simulink library "svm_lib"  (Simulink 8.6)
settings: Solver=VariableStepAuto  StartTime=0.0  StopTime=10.0  RelTol=1e-3
values from neighbouring files (symbols this model uses):
  My_3D = ([eye(6) -eye(6)])    [svm_buildLinearControllers.m]    (also in svm_setup.m = [-eye(6) eye(6)])
  turbulence2loadfactors = blkdiag(T_w2nx, T_w2nz)    [svm_buildLinearControllers.m]
  uavsim = loaded.uavsim    [svm_sandbox.m]
undefined symbols (not defined in the file or in its folder): dt, F, fflib_delay_c2d, Light, mask_p0_NED, mask_v0_NED, MIL, postracking, svm, uavsimblockset_cartesianToAngle
libraries: svm_lib x9, simulink_extras x8, aerolibtransform2 x3, formationFlyingBlockset x2, uavsimBlockset_Cularis_Aerandpropulsion x1, uavsimBlockset_ElectricPropulsion x1, aerolibwind2 x1, aerolibgravity2 x1, uavsimBlockset_VectorNorm x1, uavsimBlockset_UAV3DInterface x1
(part 2 of 3)

== system svm_lib/vector2bus u ==
  u_bus : Inport  PortDimensions=3
  Bus Object Bus Creator : BusCreator  Inputs=1  OutDataTypeStr=Bus: svm_bus_u  mask(BUS OBJECT Bus Creator){busType=Bus: svm_bus_u}
      mask prompts: busType "Bus Type"
      mask help:
      | Provides users the cabability to painlessly, instantly customize bus creators of output data type 'Bus:' by selecting the bus object type from a drop down menu dynamically populated by bus objects in the workspace.
      |
      | After pressing the "Apply Selection" button signal lines into the creator are populated and named with the elements in the chosen bus saving the user from having to recall and fill out signal line names.
      |
      | NOTE that when copying a Bus Object Bus Creator from your locked Library the link to the Library is automatically broken. This saves the user from having to Unlock Links To Library (From the Library menu.), Disable Link and finally Break Link (Both from the Model menu.) for every placed instance of the block.
      settings: AttributesFormatString=%<OutDataTypeStr>  CopyFcn=set_param(gcb, 'LinkStatus', 'none')
      mask TypeOptions busType: Bus: Acceleration | Bus: Aero | Bus: Airframe | Bus: Attitude | Bus: CMD | Bus: Environment | Bus: FlightGearData | Bus: Kinematics | Bus: Position | Bus: RotationalAcceleration | Bus: RotationalVelocity | Bus: Velocity | Bus: svm_bus_d_exo | Bus: svm_bus_u | Bus: svm_bus_x | Bus: svm_bus_xi
      mask Callback busType:
      | % Using variable names terminated with "_BOBC" to lessen the chances of
      | % collisions with existing workspace variables.
      | 
      | % Get the current block handle and mask handle.
      | handleCreator_BOBC = gcbh;
      | maskObj_BOBC       = Simulink.Mask.get(gcb);
      | 
      | % Get a list of variables in the workspace in order to search for the '1x1
      | % Bus' types.
      | wsVars_BOBC = whos;
      | 
      | % Reset the 'TypeOptions' bus list in case some '1x1 Bus' types have been
      | % deleted from or added to the workspace.
      | maskObj_BOBC.Parameters.TypeOptions = {'<empty>'};
      | 
      | % Reset the bus count.
      | busCount_BOBC = 0;
      | 
      | for index_BOBC = 1:length(wsVars_BOBC)
      | 
      |    % If the variable is a bus object...
      |    if strcmp(wsVars_BOBC(index_BOBC).class, 'Simulink.Bus')
      | 
      |       busCount_BOBC = busCount_BOBC + 1;
      | 
      |       % ... add it to the TypeOptions of the mask.
      |       maskObj_BOBC.Parameters.TypeOptions(busCount_BOBC) = ...
      |                                                            ...
      |                                  {['Bus: ', wsVars_BOBC(index_BOBC).name]};
      |    end
      | end
      | 
      | if busCount_BOBC == 0
      | 
      |    % If there are NO bus objects in the workspace then provide a warning
      |    % popup...
      |    warndlg('There are currently no bus objects in the workspace - you have no use for this block. Use a normal Bus Creator instead.')
      | 
      |    % ... and do nothing.
      | elseif ~strcmp(get_param(handleCreator_BOBC, 'OutDataTypeStr'), 'Inherit: auto')
      | 
      |    % If the currently selected bus data type ('OutDataTypeStr') is not
      |    % 'Inherit: auto' (i.e., if we are reopening the mask.) then get the
      |    % current 'OutDataTypeStr' and 'maskVal.' ('maskVal' is the selected
      |    % 'TypeOptions' list member.)
      |    outDatStr_BOBC = get_param(handleCreator_BOBC, 'OutDataTypeStr');
      |    maskVal_BOBC   = get_param(handleCreator_BOBC, 'MaskValues');
      | 
      |    if ~strcmp(outDatStr_BOBC, maskVal_BOBC{1})
      | 
      |       % Upon re-opening the mask if the default 'TypeOptions' list member
      |       % (The first one.) contained in 'maskVal' does not match the
      |       % currently selected bus data type ('OutDataTypeStr') then set the
      |       % 'TypeOptions' list member to the selected bus data type. (Cuts down
      |       % on confusion to have the displayed list member match the selected
      |       % bus data type rather than the first entry.)
      |       set_param(handleCreator_BOBC, 'MaskValues', {outDatStr_BOBC});
      |    end
      | end
      | 
      | % Clean up the workspace.
      | clear  handleCreator_BOBC  maskObj_BOBC     wsVars_BOBC ...
      |             busCount_BOBC    index_BOBC  outDatStr_BOBC ...
      |              maskVal_BOBC
      mask DialogControl applyMOCBSelection Prompt: Apply Selection
      mask DialogControl applyMOCBSelection Callback:
      | % Using variable names terminated with "_BOBC" to lessen the chances of
      | % collisions with existing workspace variables.
      | 
      | % Get the current block, current block handle and mask handle.
      | currentBlock_BOBC  = gcb;
      | handleCreator_BOBC = gcbh;
      | 
      | % Get the desired bus type...
      | desiredBusType_BOBC = get_param(handleCreator_BOBC, 'busType');
      | 
      | % ... and set the 'OutDataTypeStr' to it.
      | set_param(handleCreator_BOBC, 'OutDataTypeStr', desiredBusType_BOBC);
      | 
      | %% First delete any existing lines on the port.
      | % Get the line handles.
      | lh_BOBC = get_param(handleCreator_BOBC, 'LineHandles');
      | 
      | % If any lines exist (Non- -1 line handles.), delete them and start over.
      | if max(lh_BOBC.Inport > 0)
      | 
      |    for index_BOBC = 1:length(lh_BOBC.Inport)
      | 
      |       if lh_BOBC.Inport(index_BOBC) > 0
      | 
      |          delete_line(lh_BOBC.Inport(index_BOBC))
      |       end
      |    end
      | end
      | 
      | %% Then work on adding new lines.
      | 
      | % Get the block path for 'add_line' function.
      | blockPath_BOBC = get_param(handleCreator_BOBC, 'Parent');
      | 
      | % Get the newly selected bus type ('OutDataTypeStr')...
      | mocbBusType_BOBC = get_param(currentBlock_BOBC, 'OutDataTypeStr');
      | 
      | % ... and parse off "Bus: " so the string of the desired bus contained in
      | % 'OutDataTypeStr' matches the raw workspace bus names.
      | mocbBusType_BOBC = mocbBusType_BOBC(6:end);
      | 
      | % Then evaluate the string containing the workspace bus name which will
      | % load the desired bus parameters.
      | busParams_BOBC = eval(mocbBusType_BOBC);
      | 
      | % From the parameters grab the number of lines to add.
      | numLines_BOBC = length(busParams_BOBC.Elements);
      | 
      | % Set the number of inputs of the masked bus creator to the number of lines
      | % to add.
      | set_param(handleCreator_BOBC, 'Inputs', num2str(numLines_BOBC));
      | 
      | % Get (Inputs.) port handles so we can grab the positions of them.
      | ph_BOBC = get_param(handleCreator_BOBC, 'PortHandles');
      | 
      | for index_BOBC = 1:numLines_BOBC
      | 
      |    % Get the position of input port number 'index_BOBC'.
      |    portPos_BOBC = get_param(ph_BOBC.Inport(index_BOBC), 'Position');
      | 
      |    % Add a line from 50 pixels left of the port position to the port
      |    % position. (This must be done because it's the lines that get named,
      |    % not the port positions.)
      |    portLine_BOBC = add_line(blockPath_BOBC, [portPos_BOBC - [50 0]; portPos_BOBC]);
      | 
      |    % Rename the new line to the bus 'index_BOBC-st/nd/rd/th' element name.
      |    set_param(portLine_BOBC, 'Name', busParams_BOBC.Elements(index_BOBC).Name)
      | end
      | 
      | %% Cleanup the workspace.
      | clear    currentBlock_BOBC  handleCreator_BOBC      index_BOBC ...
      |        desiredBusType_BOBC             lh_BOBC  blockPath_BOBC ...
      |           mocbBusType_BOBC      busParams_BOBC   numLines_BOBC ...
      |                    ph_BOBC        portPos_BOBC   portLine_BOBC
  u_vector : Outport
  wires:
  u_bus/1 -> Bus Object Bus Creator/1  "n"
  Bus Object Bus Creator/1 -> u_vector/1

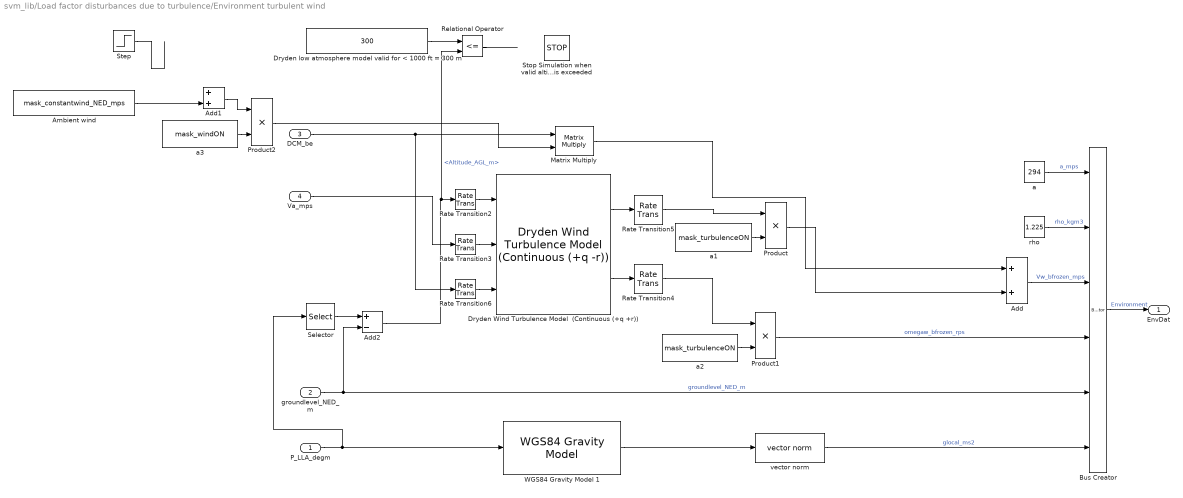
== system svm_lib/Load factor disturbances due to turbulence/Environment turbulent wind ==
  P_LLA_degm : Inport
  groundlevel_NED_m : Inport  Port=2
  DCM_be : Inport  Port=3
  Va_mps : Inport  Port=4
  Add : Sum
  Add1 : Sum
  Add2 : Sum  Inputs=+-
  Ambient wind : Constant  Value=mask_constantwind_NED_mps
  Bus Creator : BusCreator  Inputs=6  OutDataTypeStr=Bus: Environment  NonVirtualBus=on
  Dryden Wind Turbulence Model  (Continuous (+q +r)) : aerolibwind2/Dryden Wind Turbulence Model  (Continuous (+q -r))  units=Metric (MKS)  spec=MIL-F-8785C  model=Discrete Dryden (+q -r)  W20=norm(mask_constantwind_NED_mps)  Wdeg=rad2deg(uavsimblockset_cartesianToAngle(mask_constantwind_NED_mps(1), mask_constantwind_NED_mps(2)))  TurbProb=10^-2 - Light  L_high=533.4  Wingspan=mask_wingspan  ts=0.1  Seed=eval(svm.turbulenceseed)  T_on=on
  Dryden low atmosphere model valid for < 1000 ft = 300 m : Constant  Value=300
  Matrix Multiply : Product  Multiplication=Matrix(*)
  Product : Product  RndMeth=Zero
  Product1 : Product  RndMeth=Zero
  Product2 : Product  RndMeth=Zero
  Rate Transition2 : RateTransition  OutPortSampleTime=0.1
  Rate Transition3 : RateTransition  OutPortSampleTime=0.1
  Rate Transition4 : RateTransition  OutPortSampleTime=0
  Rate Transition5 : RateTransition  OutPortSampleTime=0
  Rate Transition6 : RateTransition  OutPortSampleTime=0.1
  Relational Operator : RelationalOperator  Operator=<=  OutDataTypeStr=boolean
  Selector : Selector  InputPortWidth=3  IndexOptions=Index vector (dialog)  Indices=3  OutputSizes=1
  Step : Step  Time=10  After=[0 0 1]  SampleTime=0
  Stop Simulation when valid altitude is exceeded : Stop
  WGS84 Gravity Model 1 : aerolibgravity2/WGS84 Gravity Model   model=WGS84 Taylor Series  units=Metric (MKS)  no_atmos=on  precessing=on  jd_loc=off  month=October  day=10  year=2004  no_centrifugal=on  action=Warning
  a : Constant  Value=294
  a1 : Constant  Value=mask_turbulenceON
  a2 : Constant  Value=mask_turbulenceON
  a3 : Constant  Value=mask_windON
  "rho " : Constant  Value=1.225
  vector norm : uavsimBlockset_VectorNorm/vector norm
  EnvDat : Outport  OutDataTypeStr=Bus: Environment
  wires:
  Step/1 -> ?
  Add1/1 -> Product2/1
  Product2/1 -> Matrix Multiply/2
  a3/1 -> Product2/2
  Relational Operator/1 -> ?
  Dryden low atmosphere model valid for < 1000 ft = 300 m/1 -> Relational Operator/1
  Product1/1 -> Bus Creator/4  "omegaw_bfrozen_rps"
  a2/1 -> Product1/2
  a1/1 -> Product/2
  Product/1 -> Add/2
  Dryden Wind Turbulence Model  (Continuous (+q +r))/2 -> Rate Transition4/1
  P_LLA_degm/1 -> WGS84 Gravity Model 1/1, Selector/1
  groundlevel_NED_m/1 -> Add2/2, Bus Creator/5  "groundlevel_NED_m"
  WGS84 Gravity Model 1/1 -> vector norm/1
  Bus Creator/1 -> EnvDat/1  "Environment"
  "rho "/1 -> Bus Creator/2  "rho_kgm3"
  a/1 -> Bus Creator/1  "a_mps"
  Add/1 -> Bus Creator/3  "Vw_bfrozen_mps"
  vector norm/1 -> Bus Creator/6  "glocal_ms2"
  Add2/1 -> Rate Transition2/1, Relational Operator/2  "<Altitude_AGL_m>"
  Va_mps/1 -> Rate Transition3/1
  DCM_be/1 -> Matrix Multiply/1, Rate Transition6/1
  Ambient wind/1 -> Add1/2
  Dryden Wind Turbulence Model  (Continuous (+q +r))/1 -> Rate Transition5/1
  Matrix Multiply/1 -> Add/1
  Rate Transition4/1 -> Product1/1
  Rate Transition5/1 -> Product/1
  Selector/1 -> Add2/1
  Rate Transition2/1 -> Dryden Wind Turbulence Model  (Continuous (+q +r))/1
  Rate Transition3/1 -> Dryden Wind Turbulence Model  (Continuous (+q +r))/2
  Rate Transition6/1 -> Dryden Wind Turbulence Model  (Continuous (+q +r))/3

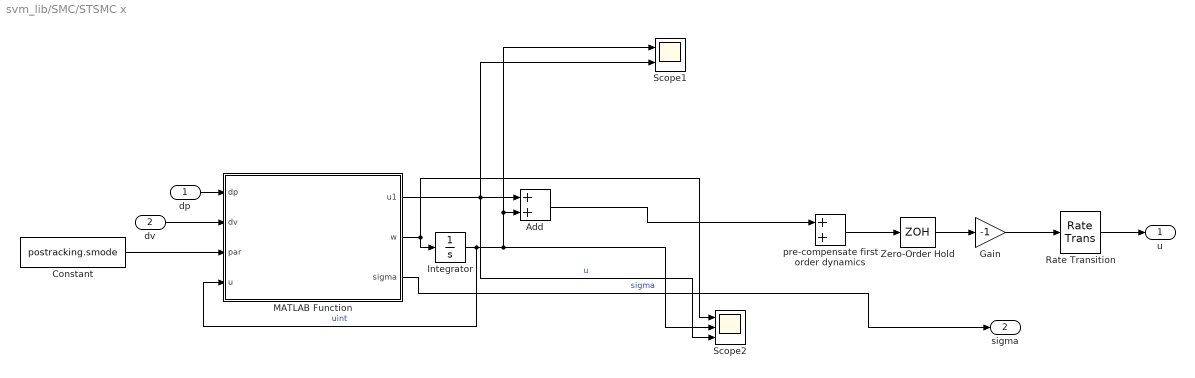
== system svm_lib/SMC/STSMC x ==
  dp : Inport
  dv : Inport  Port=2
  Add : Sum
  Constant : Constant  Value=postracking.smode  OutDataTypeStr=Bus: slBus1
  Gain : Gain  Gain=-1
  Integrator : Integrator
  MATLAB Function : MATLAB Function  TreatAsAtomicUnit=on
  Rate Transition : RateTransition
  Scope1 : Scope  NumInputPorts=2
  Scope2 : Scope  NumInputPorts=3
  Zero-Order Hold : ZeroOrderHold  SampleTime=postracking.T
  pre-compensate first order dynamics : Sum
  u : Outport  PortDimensions=1
  sigma : Outport  Port=2  PortDimensions=1
  wires:
  Gain/1 -> Rate Transition/1
  Rate Transition/1 -> u/1
  Zero-Order Hold/1 -> Gain/1
  pre-compensate first order dynamics/1 -> Zero-Order Hold/1
  MATLAB Function/2(w) -> Integrator/1, Scope2/1
  Add/1 -> pre-compensate first order dynamics/1
  Integrator/1 -> MATLAB Function/4(u), Add/2, Scope1/1, Scope2/2  "uint"
  MATLAB Function/1(u1) -> Add/1, Scope2/3, Scope1/2  "u"
  MATLAB Function/3(sigma) -> sigma/1  "sigma"
  Constant/1 -> MATLAB Function/3(par)
  dv/1 -> MATLAB Function/2(dv)
  dp/1 -> MATLAB Function/1(dp)

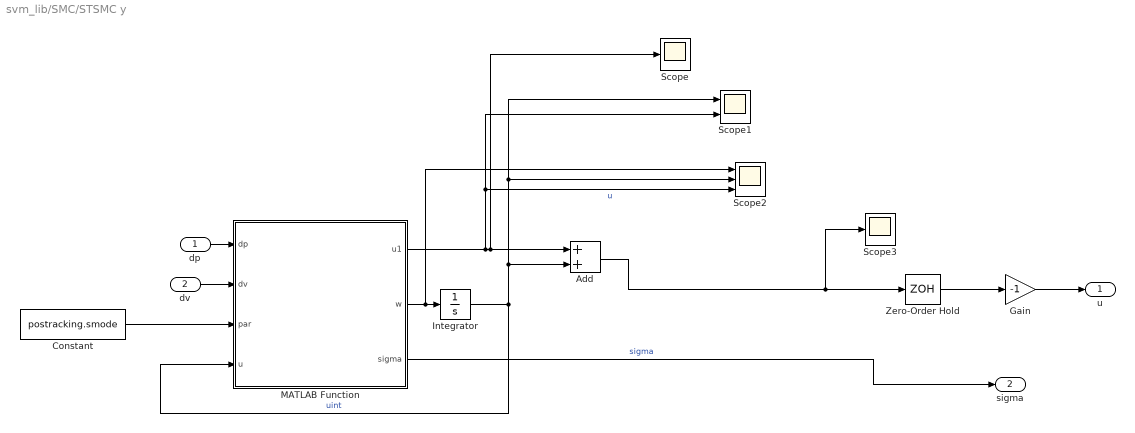
== system svm_lib/SMC/STSMC y ==
  dp : Inport
  dv : Inport  Port=2
  Add : Sum
  Constant : Constant  Value=postracking.smode  OutDataTypeStr=Bus: slBus1
  Gain : Gain  Gain=-1
  Integrator : Integrator
  MATLAB Function : MATLAB Function  TreatAsAtomicUnit=on
  Scope : Scope
  Scope1 : Scope  NumInputPorts=2
  Scope2 : Scope  NumInputPorts=3
  Scope3 : Scope
  Zero-Order Hold : ZeroOrderHold  SampleTime=postracking.T
  u : Outport  PortDimensions=1
  sigma : Outport  Port=2  PortDimensions=1
  wires:
  dp/1 -> MATLAB Function/1(dp)
  dv/1 -> MATLAB Function/2(dv)
  Constant/1 -> MATLAB Function/3(par)
  MATLAB Function/3(sigma) -> sigma/1  "sigma"
  MATLAB Function/1(u1) -> Add/1, Scope/1, Scope1/2, Scope2/3  "u"
  Integrator/1 -> MATLAB Function/4(u), Add/2, Scope1/1, Scope2/2  "uint"
  MATLAB Function/2(w) -> Integrator/1, Scope2/1
  Add/1 -> Zero-Order Hold/1, Scope3/1
  Zero-Order Hold/1 -> Gain/1
  Gain/1 -> u/1

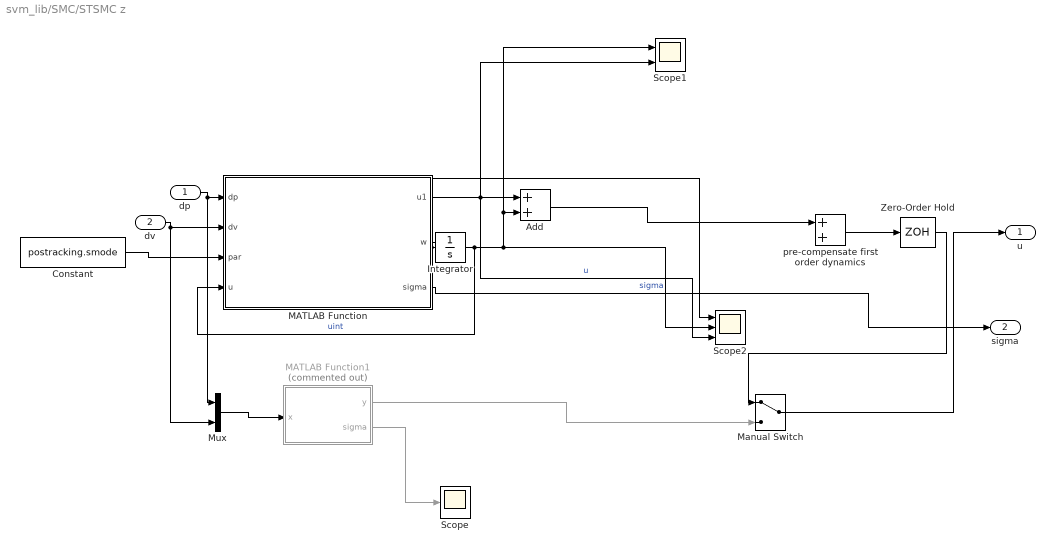
== system svm_lib/SMC/STSMC z ==
  dp : Inport
  dv : Inport  Port=2
  Add : Sum
  Constant : Constant  Value=postracking.smode  OutDataTypeStr=Bus: slBus1
  Integrator : Integrator
  MATLAB Function : MATLAB Function  TreatAsAtomicUnit=on
  MATLAB Function1 : MATLAB Function  Commented=on  TreatAsAtomicUnit=on  SystemSampleTime=dt
  Manual Switch : ManualSwitch
  Mux : Mux  Inputs=2
  Scope : Scope
  Scope1 : Scope  NumInputPorts=2
  Scope2 : Scope  NumInputPorts=3
  Zero-Order Hold : ZeroOrderHold  SampleTime=postracking.T
  pre-compensate first order dynamics : Sum
  u : Outport  PortDimensions=1
  sigma : Outport  Port=2  PortDimensions=1
  wires:
  MATLAB Function1/1(y) -> Manual Switch/2
  Zero-Order Hold/1 -> Manual Switch/1
  MATLAB Function1/2(sigma) -> Scope/1
  Mux/1 -> MATLAB Function1/1(x)
  dp/1 -> MATLAB Function/1(dp), Mux/1
  dv/1 -> MATLAB Function/2(dv), Mux/2
  Constant/1 -> MATLAB Function/3(par)
  MATLAB Function/3(sigma) -> sigma/1  "sigma"
  MATLAB Function/1(u1) -> Scope1/2, Scope2/3, Add/1  "u"
  Integrator/1 -> MATLAB Function/4(u), Scope2/2, Scope1/1, Add/2  "uint"
  Add/1 -> pre-compensate first order dynamics/1
  MATLAB Function/2(w) -> Scope2/1, Integrator/1
  pre-compensate first order dynamics/1 -> Zero-Order Hold/1
  Manual Switch/1 -> u/1

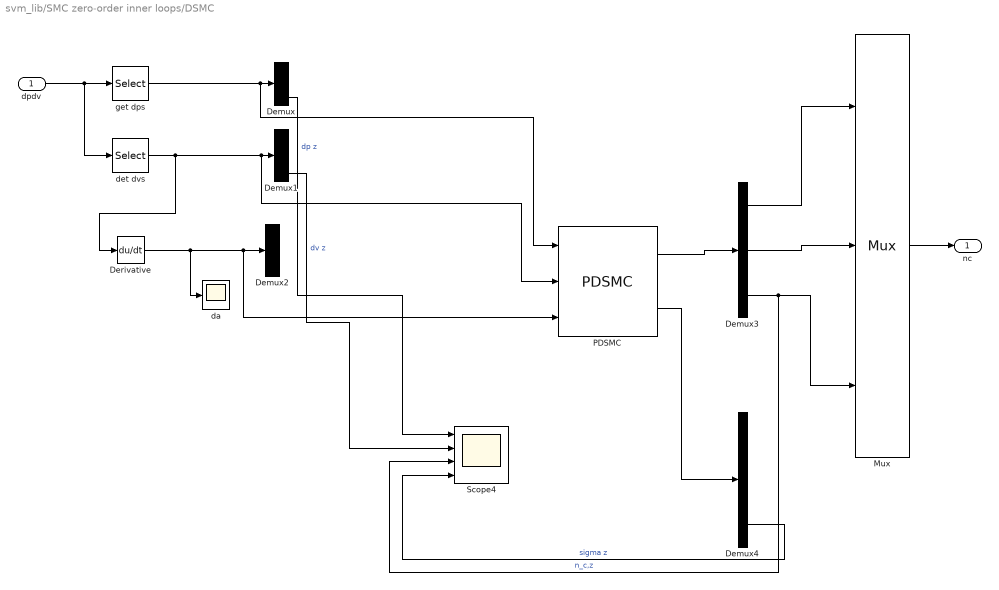
== system svm_lib/SMC zero-order inner loops/DSMC ==
  dpdv : Inport
  Demux{,1..4} (5 alike) : Demux  Outputs=3
  Derivative : Derivative
  Mux : Mux  Inputs=3
  PDSMC : svm_lib/PDSMC
  Scope4 : Scope  NumInputPorts=4
  da : Scope
  det dvs : Selector  InputPortWidth=6  IndexOptions=Index vector (dialog)  Indices=4:6  OutputSizes=1
  get dps : Selector  InputPortWidth=6  IndexOptions=Index vector (dialog)  Indices=1:3  OutputSizes=1
  nc : Outport
  wires:
  Demux/3 -> Scope4/1  "dp z"
  Demux1/3 -> Scope4/2  "dv z"
  Mux/1 -> nc/1
  get dps/1 -> PDSMC/1, Demux/1
  dpdv/1 -> get dps/1, det dvs/1
  Derivative/1 -> da/1, PDSMC/3, Demux2/1
  PDSMC/1 -> Demux3/1
  PDSMC/2 -> Demux4/1
  Demux3/3 -> Scope4/3, Mux/3  "n_c,z"
  Demux3/2 -> Mux/2
  Demux3/1 -> Mux/1
  det dvs/1 -> Derivative/1, PDSMC/2, Demux1/1
  Demux4/3 -> Scope4/4  "sigma z"

== system svm_lib/Standard Vehicle Model/Inner loop dynamics ==
  note: 1) Add Subsystem or Model blocks as valid variant choices.
      | 2) You cannot connect blocks at this level. At simulation, connectivity is automatically
      | determined, based on the active variant and port name matching.
  u : Inport
  First order models : Subsystem  VariantControl=svm_par_innerloopmode == svm_par_innerloopmodes_FORDER
  Second order models : Subsystem  VariantControl=svm_par_innerloopmode == svm_par_innerloopmodes_SORDER
  Timescale separation : Subsystem  VariantControl=svm_par_innerloopmode == svm_par_innerloopmodes_TIMESCALESEPARATION
  x_i : Outport

== system svm_lib/Standard Vehicle Model/Input saturations ==
  u : Inport  OutDataTypeStr=Bus: svm_bus_u
  Bus Selector : BusSelector  OutputSignals=n
  Bus Object Bus Creator : BusCreator  Inputs=1  OutDataTypeStr=Bus: svm_bus_u  mask(BUS OBJECT Bus Creator){busType=Bus: svm_bus_u}
      mask prompts: busType "Bus Type"
      mask help:
      | Provides users the cabability to painlessly, instantly customize bus creators of output data type 'Bus:' by selecting the bus object type from a drop down menu dynamically populated by bus objects in the workspace.
      |
      | After pressing the "Apply Selection" button signal lines into the creator are populated and named with the elements in the chosen bus saving the user from having to recall and fill out signal line names.
      |
      | NOTE that when copying a Bus Object Bus Creator from your locked Library the link to the Library is automatically broken. This saves the user from having to Unlock Links To Library (From the Library menu.), Disable Link and finally Break Link (Both from the Model menu.) for every placed instance of the block.
      settings: AttributesFormatString=%<OutDataTypeStr>  CopyFcn=set_param(gcb, 'LinkStatus', 'none')
      mask TypeOptions busType: Bus: Acceleration | Bus: Aero | Bus: Airframe | Bus: Attitude | Bus: CMD | Bus: Environment | Bus: FlightGearData | Bus: Kinematics | Bus: Position | Bus: RotationalAcceleration | Bus: RotationalVelocity | Bus: Velocity | Bus: svm_bus_d_exo | Bus: svm_bus_u | Bus: svm_bus_x | Bus: svm_bus_xi
      mask Callback busType:
      | % Using variable names terminated with "_BOBC" to lessen the chances of
      | % collisions with existing workspace variables.
      | 
      | % Get the current block handle and mask handle.
      | handleCreator_BOBC = gcbh;
      | maskObj_BOBC       = Simulink.Mask.get(gcb);
      | 
      | % Get a list of variables in the workspace in order to search for the '1x1
      | % Bus' types.
      | wsVars_BOBC = whos;
      | 
      | % Reset the 'TypeOptions' bus list in case some '1x1 Bus' types have been
      | % deleted from or added to the workspace.
      | maskObj_BOBC.Parameters.TypeOptions = {'<empty>'};
      | 
      | % Reset the bus count.
      | busCount_BOBC = 0;
      | 
      | for index_BOBC = 1:length(wsVars_BOBC)
      | 
      |    % If the variable is a bus object...
      |    if strcmp(wsVars_BOBC(index_BOBC).class, 'Simulink.Bus')
      | 
      |       busCount_BOBC = busCount_BOBC + 1;
      | 
      |       % ... add it to the TypeOptions of the mask.
      |       maskObj_BOBC.Parameters.TypeOptions(busCount_BOBC) = ...
      |                                                            ...
      |                                  {['Bus: ', wsVars_BOBC(index_BOBC).name]};
      |    end
      | end
      | 
      | if busCount_BOBC == 0
      | 
      |    % If there are NO bus objects in the workspace then provide a warning
      |    % popup...
      |    warndlg('There are currently no bus objects in the workspace - you have no use for this block. Use a normal Bus Creator instead.')
      | 
      |    % ... and do nothing.
      | elseif ~strcmp(get_param(handleCreator_BOBC, 'OutDataTypeStr'), 'Inherit: auto')
      | 
      |    % If the currently selected bus data type ('OutDataTypeStr') is not
      |    % 'Inherit: auto' (i.e., if we are reopening the mask.) then get the
      |    % current 'OutDataTypeStr' and 'maskVal.' ('maskVal' is the selected
      |    % 'TypeOptions' list member.)
      |    outDatStr_BOBC = get_param(handleCreator_BOBC, 'OutDataTypeStr');
      |    maskVal_BOBC   = get_param(handleCreator_BOBC, 'MaskValues');
      | 
      |    if ~strcmp(outDatStr_BOBC, maskVal_BOBC{1})
      | 
      |       % Upon re-opening the mask if the default 'TypeOptions' list member
      |       % (The first one.) contained in 'maskVal' does not match the
      |       % currently selected bus data type ('OutDataTypeStr') then set the
      |       % 'TypeOptions' list member to the selected bus data type. (Cuts down
      |       % on confusion to have the displayed list member match the selected
      |       % bus data type rather than the first entry.)
      |       set_param(handleCreator_BOBC, 'MaskValues', {outDatStr_BOBC});
      |    end
      | end
      | 
      | % Clean up the workspace.
      | clear  handleCreator_BOBC  maskObj_BOBC     wsVars_BOBC ...
      |             busCount_BOBC    index_BOBC  outDatStr_BOBC ...
      |              maskVal_BOBC
      mask DialogControl applyMOCBSelection Prompt: Apply Selection
      mask DialogControl applyMOCBSelection Callback:
      | % Using variable names terminated with "_BOBC" to lessen the chances of
      | % collisions with existing workspace variables.
      | 
      | % Get the current block, current block handle and mask handle.
      | currentBlock_BOBC  = gcb;
      | handleCreator_BOBC = gcbh;
      | 
      | % Get the desired bus type...
      | desiredBusType_BOBC = get_param(handleCreator_BOBC, 'busType');
      | 
      | % ... and set the 'OutDataTypeStr' to it.
      | set_param(handleCreator_BOBC, 'OutDataTypeStr', desiredBusType_BOBC);
      | 
      | %% First delete any existing lines on the port.
      | % Get the line handles.
      | lh_BOBC = get_param(handleCreator_BOBC, 'LineHandles');
      | 
      | % If any lines exist (Non- -1 line handles.), delete them and start over.
      | if max(lh_BOBC.Inport > 0)
      | 
      |    for index_BOBC = 1:length(lh_BOBC.Inport)
      | 
      |       if lh_BOBC.Inport(index_BOBC) > 0
      | 
      |          delete_line(lh_BOBC.Inport(index_BOBC))
      |       end
      |    end
      | end
      | 
      | %% Then work on adding new lines.
      | 
      | % Get the block path for 'add_line' function.
      | blockPath_BOBC = get_param(handleCreator_BOBC, 'Parent');
      | 
      | % Get the newly selected bus type ('OutDataTypeStr')...
      | mocbBusType_BOBC = get_param(currentBlock_BOBC, 'OutDataTypeStr');
      | 
      | % ... and parse off "Bus: " so the string of the desired bus contained in
      | % 'OutDataTypeStr' matches the raw workspace bus names.
      | mocbBusType_BOBC = mocbBusType_BOBC(6:end);
      | 
      | % Then evaluate the string containing the workspace bus name which will
      | % load the desired bus parameters.
      | busParams_BOBC = eval(mocbBusType_BOBC);
      | 
      | % From the parameters grab the number of lines to add.
      | numLines_BOBC = length(busParams_BOBC.Elements);
      | 
      | % Set the number of inputs of the masked bus creator to the number of lines
      | % to add.
      | set_param(handleCreator_BOBC, 'Inputs', num2str(numLines_BOBC));
      | 
      | % Get (Inputs.) port handles so we can grab the positions of them.
      | ph_BOBC = get_param(handleCreator_BOBC, 'PortHandles');
      | 
      | for index_BOBC = 1:numLines_BOBC
      | 
      |    % Get the position of input port number 'index_BOBC'.
      |    portPos_BOBC = get_param(ph_BOBC.Inport(index_BOBC), 'Position');
      | 
      |    % Add a line from 50 pixels left of the port position to the port
      |    % position. (This must be done because it's the lines that get named,
      |    % not the port positions.)
      |    portLine_BOBC = add_line(blockPath_BOBC, [portPos_BOBC - [50 0]; portPos_BOBC]);
      | 
      |    % Rename the new line to the bus 'index_BOBC-st/nd/rd/th' element name.
      |    set_param(portLine_BOBC, 'Name', busParams_BOBC.Elements(index_BOBC).Name)
      | end
      | 
      | %% Cleanup the workspace.
      | clear    currentBlock_BOBC  handleCreator_BOBC      index_BOBC ...
      |        desiredBusType_BOBC             lh_BOBC  blockPath_BOBC ...
      |           mocbBusType_BOBC      busParams_BOBC   numLines_BOBC ...
      |                    ph_BOBC        portPos_BOBC   portLine_BOBC
  Saturation : Saturate  UpperLimit=uavsim.svm.usat.n_c.upper  LowerLimit=uavsim.svm.usat.n_c.lower
  u_sat : Outport  OutDataTypeStr=Bus: svm_bus_u
  wires:
  Saturation/1 -> Bus Object Bus Creator/1  "n"
  u/1 -> Bus Selector/1
  Bus Object Bus Creator/1 -> u_sat/1
  Bus Selector/1 -> Saturation/1  "<n>"

== system svm_lib/Standard Vehicle Model/Kinematics ==
  acc : Inport
  Bus Object Bus Creator : BusCreator  Inputs=2  OutDataTypeStr=Bus: svm_bus_x  mask(BUS OBJECT Bus Creator){busType=Bus: svm_bus_x}
      mask prompts: busType "Bus Type"
      mask help:
      | Provides users the cabability to painlessly, instantly customize bus creators of output data type 'Bus:' by selecting the bus object type from a drop down menu dynamically populated by bus objects in the workspace.
      |
      | After pressing the "Apply Selection" button signal lines into the creator are populated and named with the elements in the chosen bus saving the user from having to recall and fill out signal line names.
      |
      | NOTE that when copying a Bus Object Bus Creator from your locked Library the link to the Library is automatically broken. This saves the user from having to Unlock Links To Library (From the Library menu.), Disable Link and finally Break Link (Both from the Model menu.) for every placed instance of the block.
      settings: AttributesFormatString=%<OutDataTypeStr>  CopyFcn=set_param(gcb, 'LinkStatus', 'none')
      mask TypeOptions busType: Bus: Acceleration | Bus: Aero | Bus: Airframe | Bus: Attitude | Bus: CMD | Bus: Environment | Bus: FlightGearData | Bus: Kinematics | Bus: Position | Bus: RotationalAcceleration | Bus: RotationalVelocity | Bus: Velocity | Bus: svm_bus_d_exo | Bus: svm_bus_u | Bus: svm_bus_x | Bus: svm_bus_xi
      mask Callback busType:
      | % Using variable names terminated with "_BOBC" to lessen the chances of
      | % collisions with existing workspace variables.
      | 
      | % Get the current block handle and mask handle.
      | handleCreator_BOBC = gcbh;
      | maskObj_BOBC       = Simulink.Mask.get(gcb);
      | 
      | % Get a list of variables in the workspace in order to search for the '1x1
      | % Bus' types.
      | wsVars_BOBC = whos;
      | 
      | % Reset the 'TypeOptions' bus list in case some '1x1 Bus' types have been
      | % deleted from or added to the workspace.
      | maskObj_BOBC.Parameters.TypeOptions = {'<empty>'};
      | 
      | % Reset the bus count.
      | busCount_BOBC = 0;
      | 
      | for index_BOBC = 1:length(wsVars_BOBC)
      | 
      |    % If the variable is a bus object...
      |    if strcmp(wsVars_BOBC(index_BOBC).class, 'Simulink.Bus')
      | 
      |       busCount_BOBC = busCount_BOBC + 1;
      | 
      |       % ... add it to the TypeOptions of the mask.
      |       maskObj_BOBC.Parameters.TypeOptions(busCount_BOBC) = ...
      |                                                            ...
      |                                  {['Bus: ', wsVars_BOBC(index_BOBC).name]};
      |    end
      | end
      | 
      | if busCount_BOBC == 0
      | 
      |    % If there are NO bus objects in the workspace then provide a warning
      |    % popup...
      |    warndlg('There are currently no bus objects in the workspace - you have no use for this block. Use a normal Bus Creator instead.')
      | 
      |    % ... and do nothing.
      | elseif ~strcmp(get_param(handleCreator_BOBC, 'OutDataTypeStr'), 'Inherit: auto')
      | 
      |    % If the currently selected bus data type ('OutDataTypeStr') is not
      |    % 'Inherit: auto' (i.e., if we are reopening the mask.) then get the
      |    % current 'OutDataTypeStr' and 'maskVal.' ('maskVal' is the selected
      |    % 'TypeOptions' list member.)
      |    outDatStr_BOBC = get_param(handleCreator_BOBC, 'OutDataTypeStr');
      |    maskVal_BOBC   = get_param(handleCreator_BOBC, 'MaskValues');
      | 
      |    if ~strcmp(outDatStr_BOBC, maskVal_BOBC{1})
      | 
      |       % Upon re-opening the mask if the default 'TypeOptions' list member
      |       % (The first one.) contained in 'maskVal' does not match the
      |       % currently selected bus data type ('OutDataTypeStr') then set the
      |       % 'TypeOptions' list member to the selected bus data type. (Cuts down
      |       % on confusion to have the displayed list member match the selected
      |       % bus data type rather than the first entry.)
      |       set_param(handleCreator_BOBC, 'MaskValues', {outDatStr_BOBC});
      |    end
      | end
      | 
      | % Clean up the workspace.
      | clear  handleCreator_BOBC  maskObj_BOBC     wsVars_BOBC ...
      |             busCount_BOBC    index_BOBC  outDatStr_BOBC ...
      |              maskVal_BOBC
      mask DialogControl applyMOCBSelection Prompt: Apply Selection
      mask DialogControl applyMOCBSelection Callback:
      | % Using variable names terminated with "_BOBC" to lessen the chances of
      | % collisions with existing workspace variables.
      | 
      | % Get the current block, current block handle and mask handle.
      | currentBlock_BOBC  = gcb;
      | handleCreator_BOBC = gcbh;
      | 
      | % Get the desired bus type...
      | desiredBusType_BOBC = get_param(handleCreator_BOBC, 'busType');
      | 
      | % ... and set the 'OutDataTypeStr' to it.
      | set_param(handleCreator_BOBC, 'OutDataTypeStr', desiredBusType_BOBC);
      | 
      | %% First delete any existing lines on the port.
      | % Get the line handles.
      | lh_BOBC = get_param(handleCreator_BOBC, 'LineHandles');
      | 
      | % If any lines exist (Non- -1 line handles.), delete them and start over.
      | if max(lh_BOBC.Inport > 0)
      | 
      |    for index_BOBC = 1:length(lh_BOBC.Inport)
      | 
      |       if lh_BOBC.Inport(index_BOBC) > 0
      | 
      |          delete_line(lh_BOBC.Inport(index_BOBC))
      |       end
      |    end
      | end
      | 
      | %% Then work on adding new lines.
      | 
      | % Get the block path for 'add_line' function.
      | blockPath_BOBC = get_param(handleCreator_BOBC, 'Parent');
      | 
      | % Get the newly selected bus type ('OutDataTypeStr')...
      | mocbBusType_BOBC = get_param(currentBlock_BOBC, 'OutDataTypeStr');
      | 
      | % ... and parse off "Bus: " so the string of the desired bus contained in
      | % 'OutDataTypeStr' matches the raw workspace bus names.
      | mocbBusType_BOBC = mocbBusType_BOBC(6:end);
      | 
      | % Then evaluate the string containing the workspace bus name which will
      | % load the desired bus parameters.
      | busParams_BOBC = eval(mocbBusType_BOBC);
      | 
      | % From the parameters grab the number of lines to add.
      | numLines_BOBC = length(busParams_BOBC.Elements);
      | 
      | % Set the number of inputs of the masked bus creator to the number of lines
      | % to add.
      | set_param(handleCreator_BOBC, 'Inputs', num2str(numLines_BOBC));
      | 
      | % Get (Inputs.) port handles so we can grab the positions of them.
      | ph_BOBC = get_param(handleCreator_BOBC, 'PortHandles');
      | 
      | for index_BOBC = 1:numLines_BOBC
      | 
      |    % Get the position of input port number 'index_BOBC'.
      |    portPos_BOBC = get_param(ph_BOBC.Inport(index_BOBC), 'Position');
      | 
      |    % Add a line from 50 pixels left of the port position to the port
      |    % position. (This must be done because it's the lines that get named,
      |    % not the port positions.)
      |    portLine_BOBC = add_line(blockPath_BOBC, [portPos_BOBC - [50 0]; portPos_BOBC]);
      | 
      |    % Rename the new line to the bus 'index_BOBC-st/nd/rd/th' element name.
      |    set_param(portLine_BOBC, 'Name', busParams_BOBC.Elements(index_BOBC).Name)
      | end
      | 
      | %% Cleanup the workspace.
      | clear    currentBlock_BOBC  handleCreator_BOBC      index_BOBC ...
      |        desiredBusType_BOBC             lh_BOBC  blockPath_BOBC ...
      |           mocbBusType_BOBC      busParams_BOBC   numLines_BOBC ...
      |                    ph_BOBC        portPos_BOBC   portLine_BOBC
  Sum : Sum  Inputs=|++
  p : Integrator  InitialCondition=mask_p0_NED
  v : Integrator  InitialCondition=mask_v0_NED
  x : Outport  OutDataTypeStr=Bus: svm_bus_x
  wires:
  Sum/1 -> v/1  "a_total"
  acc/1 -> Sum/1  "a_aero"
  p/1 -> Bus Object Bus Creator/1  "p"
  Bus Object Bus Creator/1 -> x/1
  v/1 -> Bus Object Bus Creator/2, p/1  "v"

== system svm_lib/Standard Vehicle Model/load factors to accelerations ==
  n : Inport
  conversion : Gain  Gain=uavsim.svm.constants.loadfactors2accelerations  Multiplication=Matrix(K*u)
  acc_mps2 : Outport
  wires:
  conversion/1 -> acc_mps2/1
  n/1 -> conversion/1

== system svm_lib/UAS 1/Controllers ==
  y : Inport
  DSMC : svm_lib/SMC zero-order inner loops/DSMC
  Form feedbacks : Gain  Gain=My_3D  Multiplication=Matrix(K*u)
  Selector : Selector  InputPortWidth=6  IndexOptions=Index vector (dialog)  Indices=1:3  OutputSizes=1
  nc : Outport
  dp : Outport  Port=2
  wires:
  Selector/1 -> dp/1
  DSMC/1 -> nc/1
  y/1 -> Form feedbacks/1
  Form feedbacks/1 -> DSMC/1, Selector/1

== system svm_lib/UAS 1/UAV3D follower ==
  x : Inport
  Bus Selector5 : BusSelector  OutputSignals=p,v
  Rate Transition10 : RateTransition  OutPortSampleTime=uavsim.svm.tsample_uav3d
  Rate Transition9 : RateTransition  OutPortSampleTime=uavsim.svm.tsample_uav3d
  Vehicle ID2 : Constant  Value=mask_vehicleID
  Visualize NED position2 : formationFlyingBlockset/Visualize leader  mask_3dmodel=1
  wires:
  x/1 -> Bus Selector5/1
  Bus Selector5/2 -> Rate Transition10/1  "<v>"
  Vehicle ID2/1 -> Visualize NED position2/3
  Bus Selector5/1 -> Rate Transition9/1  "<p>"
  Rate Transition10/1 -> Visualize NED position2/2
  Rate Transition9/1 -> Visualize NED position2/1

== system svm_lib/UAS 1/UAV3D predecessor ==
  x : Inport
  Bus Selector1 : BusSelector  OutputSignals=p,v
  Constant5 : Constant  Value=100 + mask_vehicleID
  Rate Transition5 : RateTransition  OutPortSampleTime=uavsim.svm.tsample_uav3d
  Rate Transition6 : RateTransition  OutPortSampleTime=uavsim.svm.tsample_uav3d
  Visualize NED position1 : formationFlyingBlockset/Visualize leader  mask_3dmodel=1
  wires:
  x/1 -> Bus Selector1/1
  Rate Transition5/1 -> Visualize NED position1/1
  Constant5/1 -> Visualize NED position1/3
  Rate Transition6/1 -> Visualize NED position1/2
  Bus Selector1/1 -> Rate Transition5/1  "<p>"
  Bus Selector1/2 -> Rate Transition6/1  "<v>"

== system svm_lib/Standard Vehicle Model/Inner loop dynamics/First order models ==
  u : Inport
  Bus Selector : BusSelector  OutputSignals=n
  Bus Object Bus Creator : BusCreator  Inputs=2  OutDataTypeStr=Bus: svm_bus_xi  mask(BUS OBJECT Bus Creator){busType=Bus: svm_bus_xi}
      mask prompts: busType "Bus Type"
      mask help:
      | Provides users the cabability to painlessly, instantly customize bus creators of output data type 'Bus:' by selecting the bus object type from a drop down menu dynamically populated by bus objects in the workspace.
      |
      | After pressing the "Apply Selection" button signal lines into the creator are populated and named with the elements in the chosen bus saving the user from having to recall and fill out signal line names.
      |
      | NOTE that when copying a Bus Object Bus Creator from your locked Library the link to the Library is automatically broken. This saves the user from having to Unlock Links To Library (From the Library menu.), Disable Link and finally Break Link (Both from the Model menu.) for every placed instance of the block.
      settings: AttributesFormatString=%<OutDataTypeStr>  CopyFcn=set_param(gcb, 'LinkStatus', 'none')
      mask TypeOptions busType: Bus: AHRS | Bus: Acceleration | Bus: Aero | Bus: Airdata | Bus: Airframe | Bus: Attitude | Bus: CMD | Bus: CMD_quadrotor | Bus: ControlInfoBus | Bus: Enginedata | Bus: Environment | Bus: FlightGearData | Bus: GCSUpstream | Bus: GNSSL1 | Bus: GNSSRTK | Bus: GPS | Bus: IMU | Bus: Kinematics | Bus: LandinggearInput | Bus: MotionTracker | Bus: Position | Bus: Radiodistance | Bus: RotationalAcceleration | Bus: RotationalVelocity | Bus: SensorBus | Bus: StateBus | Bus: Velocity | Bus: WindAngles | Bus: iUAScom | Bus: svm_bus_d_exo | Bus: svm_bus_u_scaled | Bus: svm_bus_x | Bus: svm_bus_xi
      mask Callback busType:
      | % Using variable names terminated with "_BOBC" to lessen the chances of
      | % collisions with existing workspace variables.
      | 
      | % Get the current block handle and mask handle.
      | handleCreator_BOBC = gcbh;
      | maskObj_BOBC       = Simulink.Mask.get(gcb);
      | 
      | % Get a list of variables in the workspace in order to search for the '1x1
      | % Bus' types.
      | wsVars_BOBC = whos;
      | 
      | % Reset the 'TypeOptions' bus list in case some '1x1 Bus' types have been
      | % deleted from or added to the workspace.
      | maskObj_BOBC.Parameters.TypeOptions = {'<empty>'};
      | 
      | % Reset the bus count.
      | busCount_BOBC = 0;
      | 
      | for index_BOBC = 1:length(wsVars_BOBC)
      | 
      |    % If the variable is a bus object...
      |    if strcmp(wsVars_BOBC(index_BOBC).class, 'Simulink.Bus')
      | 
      |       busCount_BOBC = busCount_BOBC + 1;
      | 
      |       % ... add it to the TypeOptions of the mask.
      |       maskObj_BOBC.Parameters.TypeOptions(busCount_BOBC) = ...
      |                                                            ...
      |                                  {['Bus: ', wsVars_BOBC(index_BOBC).name]};
      |    end
      | end
      | 
      | if busCount_BOBC == 0
      | 
      |    % If there are NO bus objects in the workspace then provide a warning
      |    % popup...
      |    warndlg('There are currently no bus objects in the workspace - you have no use for this block. Use a normal Bus Creator instead.')
      | 
      |    % ... and do nothing.
      | elseif ~strcmp(get_param(handleCreator_BOBC, 'OutDataTypeStr'), 'Inherit: auto')
      | 
      |    % If the currently selected bus data type ('OutDataTypeStr') is not
      |    % 'Inherit: auto' (i.e., if we are reopening the mask.) then get the
      |    % current 'OutDataTypeStr' and 'maskVal.' ('maskVal' is the selected
      |    % 'TypeOptions' list member.)
      |    outDatStr_BOBC = get_param(handleCreator_BOBC, 'OutDataTypeStr');
      |    maskVal_BOBC   = get_param(handleCreator_BOBC, 'MaskValues');
      | 
      |    if ~strcmp(outDatStr_BOBC, maskVal_BOBC{1})
      | 
      |       % Upon re-opening the mask if the default 'TypeOptions' list member
      |       % (The first one.) contained in 'maskVal' does not match the
      |       % currently selected bus data type ('OutDataTypeStr') then set the
      |       % 'TypeOptions' list member to the selected bus data type. (Cuts down
      |       % on confusion to have the displayed list member match the selected
      |       % bus data type rather than the first entry.)
      |       set_param(handleCreator_BOBC, 'MaskValues', {outDatStr_BOBC});
      |    end
      | end
      | 
      | % Clean up the workspace.
      | clear  handleCreator_BOBC  maskObj_BOBC     wsVars_BOBC ...
      |             busCount_BOBC    index_BOBC  outDatStr_BOBC ...
      |              maskVal_BOBC
      mask DialogControl applyMOCBSelection Prompt: Apply Selection
      mask DialogControl applyMOCBSelection Callback:
      | % Using variable names terminated with "_BOBC" to lessen the chances of
      | % collisions with existing workspace variables.
      | 
      | % Get the current block, current block handle and mask handle.
      | currentBlock_BOBC  = gcb;
      | handleCreator_BOBC = gcbh;
      | 
      | % Get the desired bus type...
      | desiredBusType_BOBC = get_param(handleCreator_BOBC, 'busType');
      | 
      | % ... and set the 'OutDataTypeStr' to it.
      | set_param(handleCreator_BOBC, 'OutDataTypeStr', desiredBusType_BOBC);
      | 
      | %% First delete any existing lines on the port.
      | % Get the line handles.
      | lh_BOBC = get_param(handleCreator_BOBC, 'LineHandles');
      | 
      | % If any lines exist (Non- -1 line handles.), delete them and start over.
      | if max(lh_BOBC.Inport > 0)
      | 
      |    for index_BOBC = 1:length(lh_BOBC.Inport)
      | 
      |       if lh_BOBC.Inport(index_BOBC) > 0
      | 
      |          delete_line(lh_BOBC.Inport(index_BOBC))
      |       end
      |    end
      | end
      | 
      | %% Then work on adding new lines.
      | 
      | % Get the block path for 'add_line' function.
      | blockPath_BOBC = get_param(handleCreator_BOBC, 'Parent');
      | 
      | % Get the newly selected bus type ('OutDataTypeStr')...
      | mocbBusType_BOBC = get_param(currentBlock_BOBC, 'OutDataTypeStr');
      | 
      | % ... and parse off "Bus: " so the string of the desired bus contained in
      | % 'OutDataTypeStr' matches the raw workspace bus names.
      | mocbBusType_BOBC = mocbBusType_BOBC(6:end);
      | 
      | % Then evaluate the string containing the workspace bus name which will
      | % load the desired bus parameters.
      | busParams_BOBC = eval(mocbBusType_BOBC);
      | 
      | % From the parameters grab the number of lines to add.
      | numLines_BOBC = length(busParams_BOBC.Elements);
      | 
      | % Set the number of inputs of the masked bus creator to the number of lines
      | % to add.
      | set_param(handleCreator_BOBC, 'Inputs', num2str(numLines_BOBC));
      | 
      | % Get (Inputs.) port handles so we can grab the positions of them.
      | ph_BOBC = get_param(handleCreator_BOBC, 'PortHandles');
      | 
      | for index_BOBC = 1:numLines_BOBC
      | 
      |    % Get the position of input port number 'index_BOBC'.
      |    portPos_BOBC = get_param(ph_BOBC.Inport(index_BOBC), 'Position');
      | 
      |    % Add a line from 50 pixels left of the port position to the port
      |    % position. (This must be done because it's the lines that get named,
      |    % not the port positions.)
      |    portLine_BOBC = add_line(blockPath_BOBC, [portPos_BOBC - [50 0]; portPos_BOBC]);
      | 
      |    % Rename the new line to the bus 'index_BOBC-st/nd/rd/th' element name.
      |    set_param(portLine_BOBC, 'Name', busParams_BOBC.Elements(index_BOBC).Name)
      | end
      | 
      | %% Cleanup the workspace.
      | clear    currentBlock_BOBC  handleCreator_BOBC      index_BOBC ...
      |        desiredBusType_BOBC             lh_BOBC  blockPath_BOBC ...
      |           mocbBusType_BOBC      busParams_BOBC   numLines_BOBC ...
      |                    ph_BOBC        portPos_BOBC   portLine_BOBC
  Demux1 : Demux  Outputs=3
  Mux : Mux  Inputs=3
  Transfer Fcn (with initial outputs) : simulink_extras/Additional Linear/Transfer Fcn (with initial outputs)  N=uavsim.cularis.linearModels.eulers.ss_nz_cl_forder.num{1}  D=uavsim.cularis.linearModels.eulers.ss_nz_cl_forder.den{1}  Y0=uavsim.svm.n0(3)  U0=uavsim.svm.n0(3)
  Transfer Fcn (with initial outputs)1 : simulink_extras/Additional Linear/Transfer Fcn (with initial outputs)  N=uavsim.cularis.linearModels.eulers.ss_ny_cl_forder.num{1}  D=uavsim.cularis.linearModels.eulers.ss_ny_cl_forder.den{1}  Y0=uavsim.svm.n0(2)  U0=uavsim.svm.n0(2)
  Transfer Fcn (with initial outputs)2 : simulink_extras/Additional Linear/Transfer Fcn (with initial outputs)  N=uavsim.cularis.linearModels.eulers.ss_nx_cl_forder.num{1}  D=uavsim.cularis.linearModels.eulers.ss_nx_cl_forder.den{1}  Y0=uavsim.svm.n0(1)  U0=uavsim.svm.n0(1)
  not used : Constant  Value=zeros(3,1)
  x_i : Outport
  wires:
  Transfer Fcn (with initial outputs)/1 -> Mux/3
  Bus Object Bus Creator/1 -> x_i/1
  u/1 -> Bus Selector/1
  Mux/1 -> Bus Object Bus Creator/1  "n"
  not used/1 -> Bus Object Bus Creator/2  "ndot"
  Bus Selector/1 -> Demux1/1  "<n>"
  Demux1/3 -> Transfer Fcn (with initial outputs)/1
  Demux1/2 -> Transfer Fcn (with initial outputs)1/1
  Demux1/1 -> Transfer Fcn (with initial outputs)2/1
  Transfer Fcn (with initial outputs)2/1 -> Mux/1
  Transfer Fcn (with initial outputs)1/1 -> Mux/2
